simulink model "Robot_Manipulator_Simulink"  (R2023a)
settings: Solver=VariableStepAuto  StartTime=0.0  StopTime=10.0  RelTol=1e-3
undefined symbols (not defined in the file): A, B, C, calibration_factor, K, r, x_init
settings Model: Creator=m260477  LastModifiedBy=m260477

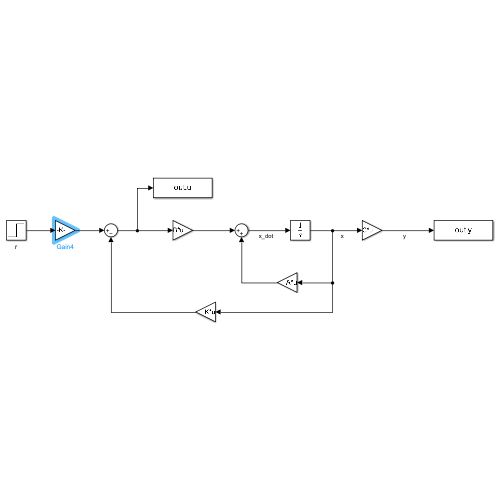
[thumbnail: Simulink's stored preview of the top-level diagram]
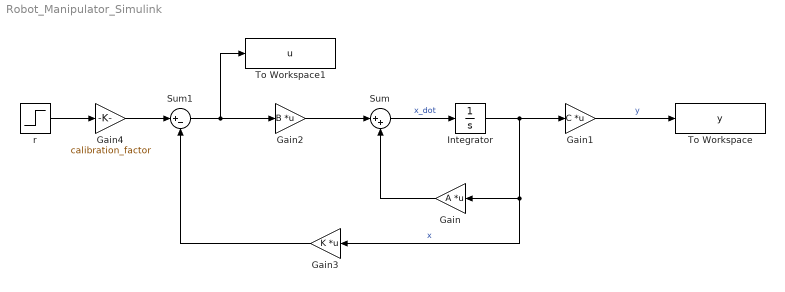
== system Robot_Manipulator_Simulink ==
  Gain : Gain  Gain=A  Multiplication=Matrix(K*u)
  Gain1 : Gain  Gain=C  Multiplication=Matrix(K*u)
  Gain2 : Gain  Gain=B  Multiplication=Matrix(K*u)
  Gain3 : Gain  Gain=K  Multiplication=Matrix(K*u)
  Gain4 : Gain  Gain=calibration_factor
  Integrator : Integrator  InitialCondition=x_init
  Sum : Sum  Inputs=|++
  Sum1 : Sum  Inputs=|+-
  To Workspace : ToWorkspace  VariableName=y  SaveFormat=Timeseries  SampleTime=-1
  To Workspace1 : ToWorkspace  VariableName=u  SaveFormat=Timeseries  SampleTime=-1
  r : Step  Time=0  After=r  SampleTime=0
  wires:
  Sum/1 -> Integrator/1  "x_dot"
  Integrator/1 -> Gain1/1, Gain3/1, Gain/1  "x"
  Gain2/1 -> Sum/1
  Gain1/1 -> To Workspace/1  "y"
  Gain/1 -> Sum/2
  Sum1/1 -> To Workspace1/1, Gain2/1
  r/1 -> Gain4/1
  Gain3/1 -> Sum1/2
  Gain4/1 -> Sum1/1
